simulink model "FirstOrderModelIC"  (R2021b)
settings: Solver=VariableStepAuto  StartTime=0.0  StopTime=50  RelTol=1e-3
undefined symbols (not defined in the file): IC, k, tau
settings Model: Creator=Jonah  LastModifiedBy=Jonah

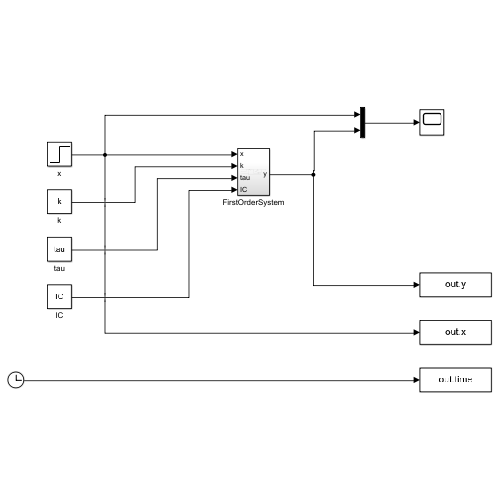
[thumbnail: Simulink's stored preview of the top-level diagram]
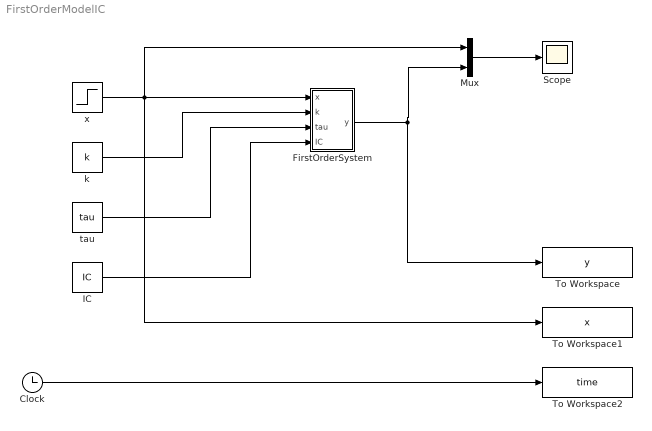
== system FirstOrderModelIC ==
  Clock : Clock
  FirstOrderSystem : Subsystem
  IC : Constant  Value=IC
  Mux : Mux  Inputs=2
  Scope : Scope
  To Workspace : ToWorkspace  VariableName=y  SampleTime=-1
  To Workspace1 : ToWorkspace  VariableName=x  SampleTime=-1
  To Workspace2 : ToWorkspace  VariableName=time  SampleTime=-1
  k : Constant  Value=k
  tau : Constant  Value=tau
  x : Step  Time=0  SampleTime=0
  wires:
  Clock/1 -> To Workspace2/1
  FirstOrderSystem/1(y) -> Mux/2, To Workspace/1
  Mux/1 -> Scope/1
  k/1 -> FirstOrderSystem/2(k)
  x/1 -> To Workspace1/1, Mux/1, FirstOrderSystem/1(x)
  tau/1 -> FirstOrderSystem/3(tau)
  IC/1 -> FirstOrderSystem/4(IC)

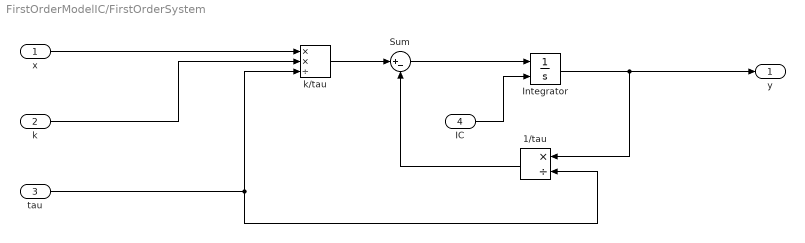
== system FirstOrderModelIC/FirstOrderSystem ==
  x : Inport
  k : Inport  Port=2
  tau : Inport  Port=3
  IC : Inport  Port=4
  1/tau : Product  Inputs=*/
  Integrator : Integrator  InitialConditionSource=external
  Sum : Sum  Inputs=|+-
  k/tau : Product  Inputs=**/
  y : Outport
  wires:
  Integrator/1 -> y/1, 1/tau/1
  tau/1 -> k/tau/3, 1/tau/2
  Sum/1 -> Integrator/1
  1/tau/1 -> Sum/2
  k/1 -> k/tau/2
  k/tau/1 -> Sum/1
  x/1 -> k/tau/1
  IC/1 -> Integrator/2
